simulink library "cal_eata"  (R2019b)
settings: Solver=VariableStepAuto  StartTime=0.0  StopTime=10.0  RelTol=1e-3
settings Model: Creator=75696  LastModifiedBy=75696

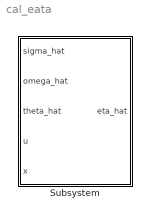
== system cal_eata ==
  Subsystem : Subsystem

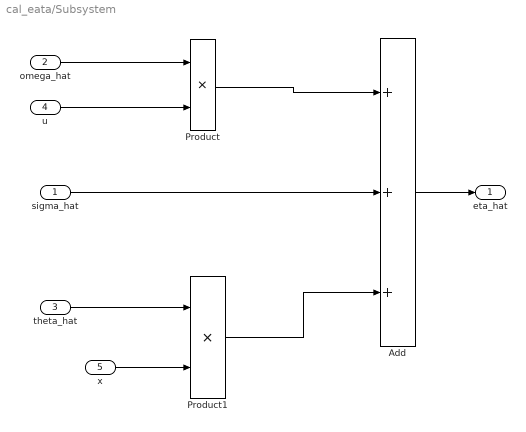
== system cal_eata/Subsystem ==
  sigma_hat : Inport
  omega_hat : Inport  Port=2
  theta_hat : Inport  Port=3
  u : Inport  Port=4
  x : Inport  Port=5
  Add : Sum  Inputs=3
  Product : Product
  Product1 : Product
  eta_hat : Outport
  wires:
  Add/1 -> eta_hat/1
  u/1 -> Product/2
  theta_hat/1 -> Product1/1
  omega_hat/1 -> Product/1
  x/1 -> Product1/2
  Product1/1 -> Add/3
  Product/1 -> Add/1
  sigma_hat/1 -> Add/2
